simulink library "AnnSoftClipperBtc"  (R2022b)
settings: Solver=VariableStepAuto  StartTime=0.0  StopTime=10.0  RelTol=1e-3
undefined symbols (not defined in the file or in its folder): Column
libraries: TuneVar x3, TOP x3, FeaturePath x1, HandyTextFile x1
settings Model: Creator=kl13806  LastModifiedBy=kl13806
settings SolverCC: AlgebraicLoopSolver=TrustRegion
settings DebuggingCC: UnconnectedInputMsg=warning  UnconnectedOutputMsg=warning  UnconnectedLineMsg=warning  SFMachineParentedDataDiag=warning
settings ModelReferenceCC: EnableRefExpFcnMdlSchedulingChecks=on
settings RTWCC: DLArmComputeVersion=19.05

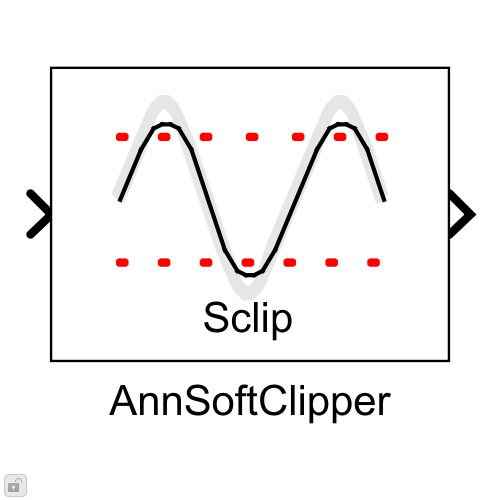
[thumbnail: Simulink's stored preview of the top-level diagram]
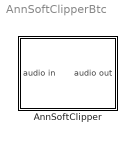
== system AnnSoftClipperBtc ==
  AnnSoftClipper : Subsystem  mask(Blocklib AnnSoftClipper){Config=[], FeatureName=Sclip}
      mask prompts: Config "AnnSoftClipperConfig"; FeatureName "Feature path name:"
      mask init:
      | blkh=gcbh;
      | Config=BTConfig.Assert(blkh,Config);
      | 
      | Config.Validate();
      | BTConfig.InitSetFeatureIfPresent(blkh,'FeatureName');
      mask Callback Config: BTConfig.CallbackHideIfPresent(gcbh,{'FeatureName'});
      mask TypeOptions FeatureName: FeaturePath/FeatureName
      mask Display:
      | [path,w,h] = IconSoftclipperMask();
      | 
      | % work in pixels since the icon does not scale
      | pos = get(gcbh,'position');
      | bw = pos(3) - pos(1);
      | bh = pos(4) - pos(2);
      | 
      | % Draw centered icon
      | xAdj = bw/2 - w/2;
      | yAdj = bh/2 - h/2 + 4;
      | for i=1:length(path)
      |     if (path(i).rgb(1) >= 0)
      |         patch(path(i).x+xAdj, path(i).y+yAdj, path(i).rgb);
      |     end
      |     if (path(i).stroke(1) >= 0)
      |         plot(path(i).x+xAdj, path(i).y+yAdj);
      |     end
      | end
      | 
      | % Anchor the corners of the coordinate system
      | patch(0,0,[1 1 1]);
      | patch(bw,bh,[1 1 1]);
      | 
      | % Display some text
      | text(bw/2, 4,FeatureName, ...
      |     'horizontalAlignment','center', ...
      |     'VerticalAlignment','bottom');

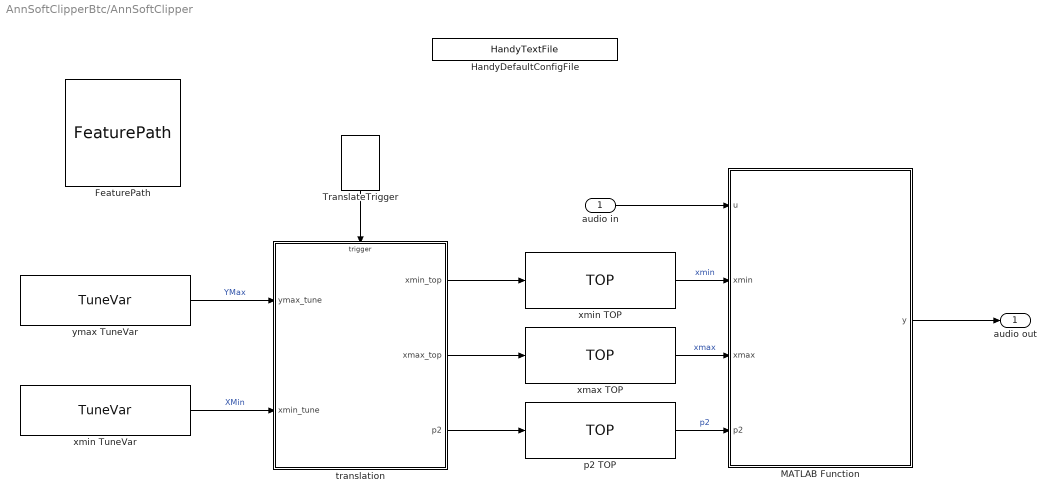
== system AnnSoftClipperBtc/AnnSoftClipper ==
  audio in : Inport
  FeaturePath : FeaturePath/FeaturePath  FeatureName=Sclip  IsGroup=off  GroupNumber=-1  IsModule=off  TriggerInit=[65 -76 180 31]
      settings: SourceProductName=Bose Talaria
  HandyDefaultConfigFile : HandyTextFile/HandyTextFile  TemplateSource=Config  FileSuffix=Init  OpenDialogOnLoad=off  UseThisBlockName=off  AddGrandParentNamePrefix=off  TheDefaultText=|  ShowInLibBrowser=on
      | % $(FILENAME) Setup model parameters for each "Init" callback (e.g. update diagram)
      | sample_rate_in_hertz = 44100;
      | frame_size = 32;
      | sysin_channel_count = 2;
      settings: SourceProductName=Bose Talaria
  MATLAB Function : MATLAB Function  TreatAsAtomicUnit=on
  TranslateTrigger : TuneVar/TranslateTrigger  TriggerInit=[341 -20 379 35]
      settings: SourceProductName=Bose Talaria
  p2 TOP : TOP/TOP  TriggerInit=[525 247 675 303]  TopName=p2  DataType=single  BankNumber=0  PreOverlay=false  PostOverlay=false  Role=Automatic
      settings: SourceProductName=Bose Talaria
  translation : MATLAB Function  TreatAsAtomicUnit=on
  xmax TOP : TOP/TOP  TriggerInit=[525 172 675 228]  TopName=xmax  DataType=single  BankNumber=0  PreOverlay=false  PostOverlay=false  Role=Automatic
      settings: SourceProductName=Bose Talaria
  xmin TOP : TOP/TOP  TriggerInit=[525 97 675 153]  TopName=xmin  DataType=single  BankNumber=0  PreOverlay=false  PostOverlay=false  Role=Automatic
      settings: SourceProductName=Bose Talaria
  xmin TuneVar : TuneVar/TuneVar  TuneName=XMin  SpecifyMaxSize=off  VariableDim=2 (Column)  MaxSize=[1 1]  TunabilityNumber=1  MinValue=[]  MaxValue=[]  TriggerInit=[20 230 190 280]  MaskValue=Config.MaskXMin
      settings: SourceProductName=Bose Talaria
  ymax TuneVar : TuneVar/TuneVar  TuneName=YMax  SpecifyMaxSize=off  VariableDim=2 (Column)  MaxSize=[1 1]  TunabilityNumber=1  MinValue=[]  MaxValue=[]  TriggerInit=[20 120 190 170]  MaskValue=Config.MaskYMax
      settings: SourceProductName=Bose Talaria
  audio out : Outport  VectorParamsAs1DForOutWhenUnconnected=off
  wires:
  audio in/1 -> MATLAB Function/1(u)
  MATLAB Function/1(y) -> audio out/1
  xmin TOP/1 -> MATLAB Function/2(xmin)  "xmin"
  xmax TOP/1 -> MATLAB Function/3(xmax)  "xmax"
  p2 TOP/1 -> MATLAB Function/4(p2)  "p2"
  translation/1(xmin_top) -> xmin TOP/1
  translation/2(xmax_top) -> xmax TOP/1
  translation/3(p2) -> p2 TOP/1
  ymax TuneVar/1 -> translation/1(ymax_tune)  "YMax"
  xmin TuneVar/1 -> translation/2(xmin_tune)  "XMin"
  TranslateTrigger/1 -> translation/Trigger

== matlab function AnnSoftClipperBtc/AnnSoftClipper/translation ==
  data: ymax_tune input; xmin_top output; xmin_tune input; xmax_top output; p2 output
  events: trigger input FUNCTION_CALL_EVENT
function [xmin_top,xmax_top, p2] = fcn(ymax_tune, xmin_tune)
% Compute the xmin and xmax value
xmin_top = xmin_tune.Value;
xmax_top = 2 * ymax_tune.Value - xmin_top;
% Compute p2
p2 = 0;
if (xmax_top ~= xmin_top)
    p2 = 1 / (2 * (xmax_top - xmin_top));
end

== matlab function AnnSoftClipperBtc/AnnSoftClipper/MATLAB Function ==
  data: u input; y output; xmin input; xmax input; p2 input
function y = softclip(u, xmin, xmax, p2)
% Grab data from input
y = coder.nullcopy(u);
[frame_size, channel_count] = size(u);
% Process the audio
for i = 1:channel_count
    for j = 1:frame_size
        % Compute the gain for this sample. Implementation copied from BDSP
        x1 = abs( u(j,i) );
        % Compute the min among x1 & xmax
        x1 = min(x1, xmax);
        x2 = x1 - xmin;
        % Compute the max among x2 and zero
        x2 = max(x2, single(0));
        x2 = x2 * x2;
        x2 = x2 * p2;
        x1 = x1 - x2;
        % Copy the sign of x1 to u
        y(j,i) = copysignf(x1, u(j,i));
    end
end
